simulink library "AEMS_Standard_Library"  (R2016b)
settings: Solver=ode45  StartTime=0.0  StopTime=10.0  RelTol=1e-3
undefined symbols (not defined in the file or in its folder): BkPY, carto, Cbx_extegr, Cbx_lpegrsys, Cbx_portegr, Cnx_bnk_nr_conf, Cnx_cyl_nr_conf, ConfigManagement, configuration_management, Cxx_dcm_io_tmr_end_xxxx, Cxx_dcm_rt_tmr_end, Cxx_DID_xxxx_IO_max, Cxx_DID_xxxx_IO_min, Cxx_egrhsofs, Cxx_vmaniegi, DEM_DEBOUNCE_FREEZE, DEM_DTR_CTL_INVISIBLE, DEM_DTR_CTL_NORMAL, Dem_DtrId2_XXX, Dem_DtrId3_XXX, Dem_DtrId4_XXX, Dem_DtrId5_XXX, Dem_DtrId6_XXX, Dem_DtrId7_XXX, Dem_DtrId8_XXX, Dem_DtrId9_XXX, Dem_DtrId_XXX, Dem_EnableConditionId2_XXX, Dem_EnableConditionId3_XXX, Dem_EnableConditionId4_XXX, Dem_EnableConditionId5_XXX, Dem_EnableConditionId6_XXX, Dem_EnableConditionId7_XXX, Dem_EnableConditionId8_XXX, Dem_EnableConditionId_XXX, Dem_EventId, Dem_EventId2_XXX, Dem_EventId3_XXX, Dem_EventId4_XXX, Dem_EventId5_XXX, Dem_EventId6_XXX, Dem_EventId7_XXX, Dem_EventId8_XXX, Dem_EventId9_XXX, Dem_EventId_Device_Faulttype, Dem_EventId_XXX, DEM_IUMPR_GENERAL_DENOMINATOR, DEM_OPCYC_IGNITION, Dem_RatioId2_XXX, Dem_RatioId3_XXX, Dem_RatioId4_XXX, Dem_RatioId5_XXX, Dem_RatioId6_XXX, Dem_RatioId7_XXX, Dem_RatioId8_XXX, Dem_RatioId_XXX, Dem_StorageConditionId2_XXX, Dem_StorageConditionId3_XXX, Dem_StorageConditionId4_XXX, Dem_StorageConditionId5_XXX ... (+65)
libraries: AEMS_Standard_Library x477, simulink x2
(part 24 of 39)

== system AEMS_Standard_Library/SUB/AEMS_DEM_SET_STORAGE_COND_8D ==
  conditionfulfilled : Inport
  AEMS_DEM_SETENABLECONDITION{1..8} (8 alike) : AEMS_Standard_Library/SUB/AEMS_DEM_SETENABLECONDITION  Tag=[LIB]
      settings: AttributesFormatString=%<MaskType>
  Demux2 : Demux  Outputs=8
  StorageConditionId_block1 : Constant  Value=Dem_StorageConditionId_XXX  OutDataTypeStr=uint8
  StorageConditionId_block2 : Constant  Value=Dem_StorageConditionId2_XXX  OutDataTypeStr=uint8
  StorageConditionId_block3 : Constant  Value=Dem_StorageConditionId3_XXX  OutDataTypeStr=uint8
  StorageConditionId_block4 : Constant  Value=Dem_StorageConditionId4_XXX  OutDataTypeStr=uint8
  StorageConditionId_block5 : Constant  Value=Dem_StorageConditionId5_XXX  OutDataTypeStr=uint8
  StorageConditionId_block6 : Constant  Value=Dem_StorageConditionId6_XXX  OutDataTypeStr=uint8
  StorageConditionId_block7 : Constant  Value=Dem_StorageConditionId7_XXX  OutDataTypeStr=uint8
  StorageConditionId_block8 : Constant  Value=Dem_StorageConditionId8_XXX  OutDataTypeStr=uint8
  wires:
  conditionfulfilled/1 -> Demux2/1  "conditionfulfilled"
  StorageConditionId_block1/1 -> AEMS_DEM_SETENABLECONDITION1/1  "storageconditionid1"
  StorageConditionId_block2/1 -> AEMS_DEM_SETENABLECONDITION2/1  "storageconditionid2"
  StorageConditionId_block4/1 -> AEMS_DEM_SETENABLECONDITION4/1  "storageconditionid4"
  StorageConditionId_block5/1 -> AEMS_DEM_SETENABLECONDITION5/1  "storageconditionid5"
  StorageConditionId_block3/1 -> AEMS_DEM_SETENABLECONDITION3/1  "storageconditionid3"
  StorageConditionId_block6/1 -> AEMS_DEM_SETENABLECONDITION6/1  "storageconditionid6"
  StorageConditionId_block7/1 -> AEMS_DEM_SETENABLECONDITION7/1  "storageconditionid7"
  StorageConditionId_block8/1 -> AEMS_DEM_SETENABLECONDITION8/1  "storageconditionid8"
  Demux2/1 -> AEMS_DEM_SETENABLECONDITION1/2  "conditionfulfilled1"
  Demux2/2 -> AEMS_DEM_SETENABLECONDITION2/2  "conditionfulfilled2"
  Demux2/3 -> AEMS_DEM_SETENABLECONDITION3/2  "conditionfulfilled3"
  Demux2/4 -> AEMS_DEM_SETENABLECONDITION4/2  "conditionfulfilled4"
  Demux2/5 -> AEMS_DEM_SETENABLECONDITION5/2  "conditionfulfilled5"
  Demux2/6 -> AEMS_DEM_SETENABLECONDITION6/2  "conditionfulfilled6"
  Demux2/7 -> AEMS_DEM_SETENABLECONDITION7/2  "conditionfulfilled7"
  Demux2/8 -> AEMS_DEM_SETENABLECONDITION8/2  "conditionfulfilled8"

== system AEMS_Standard_Library/SUB/AEMS_DEM_TIMEBASEDDEBOUNCE ==
  conditionfulfilled : Inport  OutDataTypeStr=boolean
  prefailed : Inport  Port=2  OutDataTypeStr=boolean
  prepassed : Inport  Port=3  OutDataTypeStr=boolean
  behavior : Inport  Port=4  OutDataTypeStr=uint8
  failedthreshold : Inport  Port=5  OutDataTypeStr=single
  passedthreshold : Inport  Port=6  OutDataTypeStr=single
  reseteventdebounce : Inport  Port=7  OutDataTypeStr=boolean
  Dem_SetEventStatus_Call : Subsystem  TreatAsAtomicUnit=on
  Subsystem_Timer_Debounce_Call : Subsystem
  debouncevalue_for_failed : Outport
  debouncevalue_for_passed : Outport  Port=2
  failed : Outport  Port=3
  passed : Outport  Port=4
  wires:
  Subsystem_Timer_Debounce_Call/6(eventstatus) -> Dem_SetEventStatus_Call/1(event_status)
  Subsystem_Timer_Debounce_Call/5(call_seteventstatus) -> Dem_SetEventStatus_Call/Enable
  Subsystem_Timer_Debounce_Call/1(debouncevalue_for_failed) -> debouncevalue_for_failed/1
  Subsystem_Timer_Debounce_Call/2(debouncevalue_for_passed) -> debouncevalue_for_passed/1
  Subsystem_Timer_Debounce_Call/3(failed) -> failed/1
  Subsystem_Timer_Debounce_Call/4(passed) -> passed/1
  conditionfulfilled/1 -> Subsystem_Timer_Debounce_Call/1(conditionfulfilled)
  prefailed/1 -> Subsystem_Timer_Debounce_Call/2(prefailed)
  prepassed/1 -> Subsystem_Timer_Debounce_Call/3(prepassed)
  behavior/1 -> Subsystem_Timer_Debounce_Call/4(behavior)
  failedthreshold/1 -> Subsystem_Timer_Debounce_Call/5(failedthreshold)
  passedthreshold/1 -> Subsystem_Timer_Debounce_Call/6(passedthreshold)
  reseteventdebounce/1 -> Subsystem_Timer_Debounce_Call/7(reseteventdebounce)

== system AEMS_Standard_Library/SUB/AEMS_DEM_TIME_BASED_DEBOUNCE_1D ==
  note: DemDebounceBehavior
  flag_set : Inport
  conditionfulfilled : Inport  Port=2
  prefailed : Inport  Port=3
  prepassed : Inport  Port=4
  reseteventdebounce : Inport  Port=5
  AEMS_DEM_TIME_BASED_DEBOUNCE_CALL : Subsystem
  DemCounterFailedThreshold : Constant  Value=DemDebounceTimeFailedThreshold
  DemCounterPassedThreshold : Constant  Value=DemDebounceTimePassedThreshold
  DemDebounceBehavior : Constant  Value=0  OutDataTypeStr=uint8
  debouncevalue_for_failed : Outport
  debouncevalue_for_passed : Outport  Port=2
  failed : Outport  Port=3
  passed : Outport  Port=4
  wires:
  conditionfulfilled/1 -> AEMS_DEM_TIME_BASED_DEBOUNCE_CALL/1(conditionfulfilled)  "conditionfulfilled"
  prefailed/1 -> AEMS_DEM_TIME_BASED_DEBOUNCE_CALL/2(prefailed)  "prefailed"
  prepassed/1 -> AEMS_DEM_TIME_BASED_DEBOUNCE_CALL/3(prepassed)  "prepassed"
  reseteventdebounce/1 -> AEMS_DEM_TIME_BASED_DEBOUNCE_CALL/4(reseteventdebounce)  "reseteventdebounce"
  DemDebounceBehavior/1 -> AEMS_DEM_TIME_BASED_DEBOUNCE_CALL/5(DemDebounceBehavior)  "behavior"
  DemCounterFailedThreshold/1 -> AEMS_DEM_TIME_BASED_DEBOUNCE_CALL/6(DemCounterFailedThreshold)  "failedthreshold"
  DemCounterPassedThreshold/1 -> AEMS_DEM_TIME_BASED_DEBOUNCE_CALL/7(DemCounterPassedThreshold)  "passedthreshold"
  AEMS_DEM_TIME_BASED_DEBOUNCE_CALL/1(debouncevalue_for_failed) -> debouncevalue_for_failed/1
  AEMS_DEM_TIME_BASED_DEBOUNCE_CALL/2(debouncevalue_for_passed) -> debouncevalue_for_passed/1
  AEMS_DEM_TIME_BASED_DEBOUNCE_CALL/3(failed) -> failed/1
  AEMS_DEM_TIME_BASED_DEBOUNCE_CALL/4(passed) -> passed/1
  flag_set/1 -> AEMS_DEM_TIME_BASED_DEBOUNCE_CALL/Enable

== system AEMS_Standard_Library/SUB/AEMS_DEM_TIME_BASED_DEBOUNCE_2D ==
  note: DemDebounceBehavior
  flag_set : Inport
  conditionfulfilled : Inport  Port=2
  prefailed : Inport  Port=3
  prepassed : Inport  Port=4
  reseteventdebounce : Inport  Port=5
  AEMS_DEM_TIME_BASED_DEBOUNCE_CALL1 : Subsystem
  AEMS_DEM_TIME_BASED_DEBOUNCE_CALL2 : Subsystem
  DemCounterFailedThreshold : Constant  Value=DemDebounceTimeFailedThreshold
  DemCounterPassedThreshold : Constant  Value=DemDebounceTimePassedThreshold
  DemDebounceBehavior : Constant  Value=[0,0]  OutDataTypeStr=uint8
  Demux{,1..7} (8 alike) : Demux  Outputs=2
  Mux{1..4} (4 alike) : Mux  Inputs=2
  debouncevalue_for_failed : Outport
  debouncevalue_for_passed : Outport  Port=2
  failed : Outport  Port=3
  passed : Outport  Port=4
  wires:
  AEMS_DEM_TIME_BASED_DEBOUNCE_CALL2/4(passed) -> Mux4/2
  Mux4/1 -> passed/1
  AEMS_DEM_TIME_BASED_DEBOUNCE_CALL1/4(passed) -> Mux4/1
  AEMS_DEM_TIME_BASED_DEBOUNCE_CALL2/3(failed) -> Mux3/2
  AEMS_DEM_TIME_BASED_DEBOUNCE_CALL1/3(failed) -> Mux3/1
  Mux3/1 -> failed/1
  AEMS_DEM_TIME_BASED_DEBOUNCE_CALL2/2(debouncevalue_for_passed) -> Mux2/2
  AEMS_DEM_TIME_BASED_DEBOUNCE_CALL1/2(debouncevalue_for_passed) -> Mux2/1
  Mux2/1 -> debouncevalue_for_passed/1
  AEMS_DEM_TIME_BASED_DEBOUNCE_CALL2/1(debouncevalue_for_failed) -> Mux1/2
  AEMS_DEM_TIME_BASED_DEBOUNCE_CALL1/1(debouncevalue_for_failed) -> Mux1/1
  Mux1/1 -> debouncevalue_for_failed/1
  Demux7/2 -> AEMS_DEM_TIME_BASED_DEBOUNCE_CALL2/7(DemCounterPassedThreshold)
  DemCounterPassedThreshold/1 -> Demux7/1  "passedthreshold"
  Demux7/1 -> AEMS_DEM_TIME_BASED_DEBOUNCE_CALL1/7(DemCounterPassedThreshold)
  Demux6/2 -> AEMS_DEM_TIME_BASED_DEBOUNCE_CALL2/6(DemCounterFailedThreshold)
  DemCounterFailedThreshold/1 -> Demux6/1  "failedthreshold"
  Demux6/1 -> AEMS_DEM_TIME_BASED_DEBOUNCE_CALL1/6(DemCounterFailedThreshold)
  Demux5/2 -> AEMS_DEM_TIME_BASED_DEBOUNCE_CALL2/5(DemDebounceBehavior)
  Demux5/1 -> AEMS_DEM_TIME_BASED_DEBOUNCE_CALL1/5(DemDebounceBehavior)
  DemDebounceBehavior/1 -> Demux5/1  "behavior"
  Demux4/2 -> AEMS_DEM_TIME_BASED_DEBOUNCE_CALL2/4(reseteventdebounce)
  reseteventdebounce/1 -> Demux4/1  "reseteventdebounce"
  Demux4/1 -> AEMS_DEM_TIME_BASED_DEBOUNCE_CALL1/4(reseteventdebounce)
  Demux3/2 -> AEMS_DEM_TIME_BASED_DEBOUNCE_CALL2/3(prepassed)
  Demux3/1 -> AEMS_DEM_TIME_BASED_DEBOUNCE_CALL1/3(prepassed)
  prepassed/1 -> Demux3/1  "prepassed"
  Demux2/2 -> AEMS_DEM_TIME_BASED_DEBOUNCE_CALL2/2(prefailed)
  Demux2/1 -> AEMS_DEM_TIME_BASED_DEBOUNCE_CALL1/2(prefailed)
  prefailed/1 -> Demux2/1  "prefailed"
  Demux1/2 -> AEMS_DEM_TIME_BASED_DEBOUNCE_CALL2/1(conditionfulfilled)
  Demux/2 -> AEMS_DEM_TIME_BASED_DEBOUNCE_CALL2/Enable
  Demux1/1 -> AEMS_DEM_TIME_BASED_DEBOUNCE_CALL1/1(conditionfulfilled)
  conditionfulfilled/1 -> Demux1/1  "conditionfulfilled"
  Demux/1 -> AEMS_DEM_TIME_BASED_DEBOUNCE_CALL1/Enable
  flag_set/1 -> Demux/1

== system AEMS_Standard_Library/SUB/AEMS_DEM_TIME_BASED_DEBOUNCE_3D ==
  note: DemDebounceBehavior
  flag_set : Inport
  conditionfulfilled : Inport  Port=2
  prefailed : Inport  Port=3
  prepassed : Inport  Port=4
  reseteventdebounce : Inport  Port=5
  AEMS_DEM_TIME_BASED_DEBOUNCE_CALL1 : Subsystem
  AEMS_DEM_TIME_BASED_DEBOUNCE_CALL2 : Subsystem
  AEMS_DEM_TIME_BASED_DEBOUNCE_CALL3 : Subsystem
  DemCounterFailedThreshold : Constant  Value=DemDebounceTimeFailedThreshold
  DemCounterPassedThreshold : Constant  Value=DemDebounceTimePassedThreshold
  DemDebounceBehavior : Constant  Value=[0,0,0]  OutDataTypeStr=uint8
  Demux{,1..7} (8 alike) : Demux  Outputs=3
  Mux{1..4} (4 alike) : Mux  Inputs=3
  debouncevalue_for_failed : Outport
  debouncevalue_for_passed : Outport  Port=2
  failed : Outport  Port=3
  passed : Outport  Port=4
  wires:
  AEMS_DEM_TIME_BASED_DEBOUNCE_CALL3/4(passed) -> Mux4/3
  AEMS_DEM_TIME_BASED_DEBOUNCE_CALL3/3(failed) -> Mux3/3
  AEMS_DEM_TIME_BASED_DEBOUNCE_CALL3/2(debouncevalue_for_passed) -> Mux2/3
  AEMS_DEM_TIME_BASED_DEBOUNCE_CALL3/1(debouncevalue_for_failed) -> Mux1/3
  Demux7/3 -> AEMS_DEM_TIME_BASED_DEBOUNCE_CALL3/7(DemCounterPassedThreshold)
  Demux6/3 -> AEMS_DEM_TIME_BASED_DEBOUNCE_CALL3/6(DemCounterFailedThreshold)
  Demux5/3 -> AEMS_DEM_TIME_BASED_DEBOUNCE_CALL3/5(DemDebounceBehavior)
  Demux4/3 -> AEMS_DEM_TIME_BASED_DEBOUNCE_CALL3/4(reseteventdebounce)
  Demux3/3 -> AEMS_DEM_TIME_BASED_DEBOUNCE_CALL3/3(prepassed)
  Demux2/3 -> AEMS_DEM_TIME_BASED_DEBOUNCE_CALL3/2(prefailed)
  Demux1/3 -> AEMS_DEM_TIME_BASED_DEBOUNCE_CALL3/1(conditionfulfilled)
  Demux/3 -> AEMS_DEM_TIME_BASED_DEBOUNCE_CALL3/Enable
  AEMS_DEM_TIME_BASED_DEBOUNCE_CALL2/4(passed) -> Mux4/2
  Mux4/1 -> passed/1
  AEMS_DEM_TIME_BASED_DEBOUNCE_CALL1/4(passed) -> Mux4/1
  AEMS_DEM_TIME_BASED_DEBOUNCE_CALL2/3(failed) -> Mux3/2
  AEMS_DEM_TIME_BASED_DEBOUNCE_CALL1/3(failed) -> Mux3/1
  Mux3/1 -> failed/1
  AEMS_DEM_TIME_BASED_DEBOUNCE_CALL2/2(debouncevalue_for_passed) -> Mux2/2
  AEMS_DEM_TIME_BASED_DEBOUNCE_CALL1/2(debouncevalue_for_passed) -> Mux2/1
  Mux2/1 -> debouncevalue_for_passed/1
  AEMS_DEM_TIME_BASED_DEBOUNCE_CALL2/1(debouncevalue_for_failed) -> Mux1/2
  AEMS_DEM_TIME_BASED_DEBOUNCE_CALL1/1(debouncevalue_for_failed) -> Mux1/1
  Mux1/1 -> debouncevalue_for_failed/1
  Demux7/2 -> AEMS_DEM_TIME_BASED_DEBOUNCE_CALL2/7(DemCounterPassedThreshold)
  DemCounterPassedThreshold/1 -> Demux7/1  "passedthreshold"
  Demux7/1 -> AEMS_DEM_TIME_BASED_DEBOUNCE_CALL1/7(DemCounterPassedThreshold)
  Demux6/2 -> AEMS_DEM_TIME_BASED_DEBOUNCE_CALL2/6(DemCounterFailedThreshold)
  DemCounterFailedThreshold/1 -> Demux6/1  "failedthreshold"
  Demux6/1 -> AEMS_DEM_TIME_BASED_DEBOUNCE_CALL1/6(DemCounterFailedThreshold)
  Demux5/2 -> AEMS_DEM_TIME_BASED_DEBOUNCE_CALL2/5(DemDebounceBehavior)
  Demux5/1 -> AEMS_DEM_TIME_BASED_DEBOUNCE_CALL1/5(DemDebounceBehavior)
  DemDebounceBehavior/1 -> Demux5/1  "behavior"
  Demux4/2 -> AEMS_DEM_TIME_BASED_DEBOUNCE_CALL2/4(reseteventdebounce)
  reseteventdebounce/1 -> Demux4/1  "reseteventdebounce"
  Demux4/1 -> AEMS_DEM_TIME_BASED_DEBOUNCE_CALL1/4(reseteventdebounce)
  Demux3/2 -> AEMS_DEM_TIME_BASED_DEBOUNCE_CALL2/3(prepassed)
  Demux3/1 -> AEMS_DEM_TIME_BASED_DEBOUNCE_CALL1/3(prepassed)
  prepassed/1 -> Demux3/1  "prepassed"
  Demux2/2 -> AEMS_DEM_TIME_BASED_DEBOUNCE_CALL2/2(prefailed)
  Demux2/1 -> AEMS_DEM_TIME_BASED_DEBOUNCE_CALL1/2(prefailed)
  prefailed/1 -> Demux2/1  "prefailed"
  Demux1/2 -> AEMS_DEM_TIME_BASED_DEBOUNCE_CALL2/1(conditionfulfilled)
  Demux/2 -> AEMS_DEM_TIME_BASED_DEBOUNCE_CALL2/Enable
  Demux1/1 -> AEMS_DEM_TIME_BASED_DEBOUNCE_CALL1/1(conditionfulfilled)
  conditionfulfilled/1 -> Demux1/1  "conditionfulfilled"
  Demux/1 -> AEMS_DEM_TIME_BASED_DEBOUNCE_CALL1/Enable
  flag_set/1 -> Demux/1

== system AEMS_Standard_Library/SUB/AEMS_DEM_TIME_BASED_DEBOUNCE_4D ==
  note: DemDebounceBehavior
  flag_set : Inport
  conditionfulfilled : Inport  Port=2
  prefailed : Inport  Port=3
  prepassed : Inport  Port=4
  reseteventdebounce : Inport  Port=5
  AEMS_DEM_TIME_BASED_DEBOUNCE_CALL1 : Subsystem
  AEMS_DEM_TIME_BASED_DEBOUNCE_CALL2 : Subsystem
  AEMS_DEM_TIME_BASED_DEBOUNCE_CALL3 : Subsystem
  AEMS_DEM_TIME_BASED_DEBOUNCE_CALL4 : Subsystem
  DemCounterFailedThreshold : Constant  Value=DemDebounceTimeFailedThreshold
  DemCounterPassedThreshold : Constant  Value=DemDebounceTimePassedThreshold
  DemDebounceBehavior : Constant  Value=[0,0,0,0]  OutDataTypeStr=uint8
  Demux{,1..7} (8 alike) : Demux
  Mux{1..4} (4 alike) : Mux
  debouncevalue_for_failed : Outport
  debouncevalue_for_passed : Outport  Port=2
  failed : Outport  Port=3
  passed : Outport  Port=4
  wires:
  AEMS_DEM_TIME_BASED_DEBOUNCE_CALL4/4(passed) -> Mux4/4
  AEMS_DEM_TIME_BASED_DEBOUNCE_CALL4/3(failed) -> Mux3/4
  AEMS_DEM_TIME_BASED_DEBOUNCE_CALL4/2(debouncevalue_for_passed) -> Mux2/4
  AEMS_DEM_TIME_BASED_DEBOUNCE_CALL4/1(debouncevalue_for_failed) -> Mux1/4
  Demux7/4 -> AEMS_DEM_TIME_BASED_DEBOUNCE_CALL4/7(DemCounterPassedThreshold)
  Demux6/4 -> AEMS_DEM_TIME_BASED_DEBOUNCE_CALL4/6(DemCounterFailedThreshold)
  Demux5/4 -> AEMS_DEM_TIME_BASED_DEBOUNCE_CALL4/5(DemDebounceBehavior)
  Demux4/4 -> AEMS_DEM_TIME_BASED_DEBOUNCE_CALL4/4(reseteventdebounce)
  Demux3/4 -> AEMS_DEM_TIME_BASED_DEBOUNCE_CALL4/3(prepassed)
  Demux2/4 -> AEMS_DEM_TIME_BASED_DEBOUNCE_CALL4/2(prefailed)
  Demux1/4 -> AEMS_DEM_TIME_BASED_DEBOUNCE_CALL4/1(conditionfulfilled)
  Demux/4 -> AEMS_DEM_TIME_BASED_DEBOUNCE_CALL4/Enable
  AEMS_DEM_TIME_BASED_DEBOUNCE_CALL3/4(passed) -> Mux4/3
  AEMS_DEM_TIME_BASED_DEBOUNCE_CALL3/3(failed) -> Mux3/3
  AEMS_DEM_TIME_BASED_DEBOUNCE_CALL3/2(debouncevalue_for_passed) -> Mux2/3
  AEMS_DEM_TIME_BASED_DEBOUNCE_CALL3/1(debouncevalue_for_failed) -> Mux1/3
  Demux7/3 -> AEMS_DEM_TIME_BASED_DEBOUNCE_CALL3/7(DemCounterPassedThreshold)
  Demux6/3 -> AEMS_DEM_TIME_BASED_DEBOUNCE_CALL3/6(DemCounterFailedThreshold)
  Demux5/3 -> AEMS_DEM_TIME_BASED_DEBOUNCE_CALL3/5(DemDebounceBehavior)
  Demux4/3 -> AEMS_DEM_TIME_BASED_DEBOUNCE_CALL3/4(reseteventdebounce)
  Demux3/3 -> AEMS_DEM_TIME_BASED_DEBOUNCE_CALL3/3(prepassed)
  Demux2/3 -> AEMS_DEM_TIME_BASED_DEBOUNCE_CALL3/2(prefailed)
  Demux1/3 -> AEMS_DEM_TIME_BASED_DEBOUNCE_CALL3/1(conditionfulfilled)
  Demux/3 -> AEMS_DEM_TIME_BASED_DEBOUNCE_CALL3/Enable
  AEMS_DEM_TIME_BASED_DEBOUNCE_CALL2/4(passed) -> Mux4/2
  Mux4/1 -> passed/1
  AEMS_DEM_TIME_BASED_DEBOUNCE_CALL1/4(passed) -> Mux4/1
  AEMS_DEM_TIME_BASED_DEBOUNCE_CALL2/3(failed) -> Mux3/2
  AEMS_DEM_TIME_BASED_DEBOUNCE_CALL1/3(failed) -> Mux3/1
  Mux3/1 -> failed/1
  AEMS_DEM_TIME_BASED_DEBOUNCE_CALL2/2(debouncevalue_for_passed) -> Mux2/2
  AEMS_DEM_TIME_BASED_DEBOUNCE_CALL1/2(debouncevalue_for_passed) -> Mux2/1
  Mux2/1 -> debouncevalue_for_passed/1
  AEMS_DEM_TIME_BASED_DEBOUNCE_CALL2/1(debouncevalue_for_failed) -> Mux1/2
  AEMS_DEM_TIME_BASED_DEBOUNCE_CALL1/1(debouncevalue_for_failed) -> Mux1/1
  Mux1/1 -> debouncevalue_for_failed/1
  Demux7/2 -> AEMS_DEM_TIME_BASED_DEBOUNCE_CALL2/7(DemCounterPassedThreshold)
  DemCounterPassedThreshold/1 -> Demux7/1  "passedthreshold"
  Demux7/1 -> AEMS_DEM_TIME_BASED_DEBOUNCE_CALL1/7(DemCounterPassedThreshold)
  Demux6/2 -> AEMS_DEM_TIME_BASED_DEBOUNCE_CALL2/6(DemCounterFailedThreshold)
  DemCounterFailedThreshold/1 -> Demux6/1  "failedthreshold"
  Demux6/1 -> AEMS_DEM_TIME_BASED_DEBOUNCE_CALL1/6(DemCounterFailedThreshold)
  Demux5/2 -> AEMS_DEM_TIME_BASED_DEBOUNCE_CALL2/5(DemDebounceBehavior)
  Demux5/1 -> AEMS_DEM_TIME_BASED_DEBOUNCE_CALL1/5(DemDebounceBehavior)
  DemDebounceBehavior/1 -> Demux5/1  "behavior"
  Demux4/2 -> AEMS_DEM_TIME_BASED_DEBOUNCE_CALL2/4(reseteventdebounce)
  reseteventdebounce/1 -> Demux4/1  "reseteventdebounce"
  Demux4/1 -> AEMS_DEM_TIME_BASED_DEBOUNCE_CALL1/4(reseteventdebounce)
  Demux3/2 -> AEMS_DEM_TIME_BASED_DEBOUNCE_CALL2/3(prepassed)
  Demux3/1 -> AEMS_DEM_TIME_BASED_DEBOUNCE_CALL1/3(prepassed)
  prepassed/1 -> Demux3/1  "prepassed"
  Demux2/2 -> AEMS_DEM_TIME_BASED_DEBOUNCE_CALL2/2(prefailed)
  Demux2/1 -> AEMS_DEM_TIME_BASED_DEBOUNCE_CALL1/2(prefailed)
  prefailed/1 -> Demux2/1  "prefailed"
  Demux1/2 -> AEMS_DEM_TIME_BASED_DEBOUNCE_CALL2/1(conditionfulfilled)
  Demux/2 -> AEMS_DEM_TIME_BASED_DEBOUNCE_CALL2/Enable
  Demux1/1 -> AEMS_DEM_TIME_BASED_DEBOUNCE_CALL1/1(conditionfulfilled)
  conditionfulfilled/1 -> Demux1/1  "conditionfulfilled"
  Demux/1 -> AEMS_DEM_TIME_BASED_DEBOUNCE_CALL1/Enable
  flag_set/1 -> Demux/1

== system AEMS_Standard_Library/SUB/AEMS_DEM_TIME_BASED_DEBOUNCE_6D ==
  note: DemDebounceBehavior
  flag_set : Inport
  conditionfulfilled : Inport  Port=2
  prefailed : Inport  Port=3
  prepassed : Inport  Port=4
  reseteventdebounce : Inport  Port=5
  AEMS_DEM_TIME_BASED_DEBOUNCE_CALL1 : Subsystem
  AEMS_DEM_TIME_BASED_DEBOUNCE_CALL2 : Subsystem
  AEMS_DEM_TIME_BASED_DEBOUNCE_CALL3 : Subsystem
  AEMS_DEM_TIME_BASED_DEBOUNCE_CALL4 : Subsystem
  AEMS_DEM_TIME_BASED_DEBOUNCE_CALL5 : Subsystem
  AEMS_DEM_TIME_BASED_DEBOUNCE_CALL6 : Subsystem
  DemCounterFailedThreshold : Constant  Value=DemDebounceTimeFailedThreshold
  DemCounterPassedThreshold : Constant  Value=DemDebounceTimePassedThreshold
  DemDebounceBehavior : Constant  Value=[0,0,0,0,0,0]  OutDataTypeStr=uint8
  Demux{,1..7} (8 alike) : Demux  Outputs=6
  Mux{1..4} (4 alike) : Mux  Inputs=6
  debouncevalue_for_failed : Outport
  debouncevalue_for_passed : Outport  Port=2
  failed : Outport  Port=3
  passed : Outport  Port=4
  wires:
  AEMS_DEM_TIME_BASED_DEBOUNCE_CALL6/4(passed) -> Mux4/6
  AEMS_DEM_TIME_BASED_DEBOUNCE_CALL5/4(passed) -> Mux4/5
  AEMS_DEM_TIME_BASED_DEBOUNCE_CALL6/3(failed) -> Mux3/6
  AEMS_DEM_TIME_BASED_DEBOUNCE_CALL5/3(failed) -> Mux3/5
  AEMS_DEM_TIME_BASED_DEBOUNCE_CALL6/2(debouncevalue_for_passed) -> Mux2/6
  AEMS_DEM_TIME_BASED_DEBOUNCE_CALL5/2(debouncevalue_for_passed) -> Mux2/5
  AEMS_DEM_TIME_BASED_DEBOUNCE_CALL6/1(debouncevalue_for_failed) -> Mux1/6
  AEMS_DEM_TIME_BASED_DEBOUNCE_CALL5/1(debouncevalue_for_failed) -> Mux1/5
  Demux7/6 -> AEMS_DEM_TIME_BASED_DEBOUNCE_CALL6/7(DemCounterPassedThreshold)
  Demux7/5 -> AEMS_DEM_TIME_BASED_DEBOUNCE_CALL5/7(DemCounterPassedThreshold)
  Demux6/6 -> AEMS_DEM_TIME_BASED_DEBOUNCE_CALL6/6(DemCounterFailedThreshold)
  Demux6/5 -> AEMS_DEM_TIME_BASED_DEBOUNCE_CALL5/6(DemCounterFailedThreshold)
  Demux5/6 -> AEMS_DEM_TIME_BASED_DEBOUNCE_CALL6/5(DemDebounceBehavior)
  Demux5/5 -> AEMS_DEM_TIME_BASED_DEBOUNCE_CALL5/5(DemDebounceBehavior)
  Demux4/6 -> AEMS_DEM_TIME_BASED_DEBOUNCE_CALL6/4(reseteventdebounce)
  Demux4/5 -> AEMS_DEM_TIME_BASED_DEBOUNCE_CALL5/4(reseteventdebounce)
  Demux3/6 -> AEMS_DEM_TIME_BASED_DEBOUNCE_CALL6/3(prepassed)
  Demux3/5 -> AEMS_DEM_TIME_BASED_DEBOUNCE_CALL5/3(prepassed)
  Demux2/6 -> AEMS_DEM_TIME_BASED_DEBOUNCE_CALL6/2(prefailed)
  Demux2/5 -> AEMS_DEM_TIME_BASED_DEBOUNCE_CALL5/2(prefailed)
  Demux1/6 -> AEMS_DEM_TIME_BASED_DEBOUNCE_CALL6/1(conditionfulfilled)
  Demux1/5 -> AEMS_DEM_TIME_BASED_DEBOUNCE_CALL5/1(conditionfulfilled)
  Demux/6 -> AEMS_DEM_TIME_BASED_DEBOUNCE_CALL6/Enable
  Demux/5 -> AEMS_DEM_TIME_BASED_DEBOUNCE_CALL5/Enable
  AEMS_DEM_TIME_BASED_DEBOUNCE_CALL4/4(passed) -> Mux4/4
  AEMS_DEM_TIME_BASED_DEBOUNCE_CALL4/3(failed) -> Mux3/4
  AEMS_DEM_TIME_BASED_DEBOUNCE_CALL4/2(debouncevalue_for_passed) -> Mux2/4
  AEMS_DEM_TIME_BASED_DEBOUNCE_CALL4/1(debouncevalue_for_failed) -> Mux1/4
  Demux7/4 -> AEMS_DEM_TIME_BASED_DEBOUNCE_CALL4/7(DemCounterPassedThreshold)
  Demux6/4 -> AEMS_DEM_TIME_BASED_DEBOUNCE_CALL4/6(DemCounterFailedThreshold)
  Demux5/4 -> AEMS_DEM_TIME_BASED_DEBOUNCE_CALL4/5(DemDebounceBehavior)
  Demux4/4 -> AEMS_DEM_TIME_BASED_DEBOUNCE_CALL4/4(reseteventdebounce)
  Demux3/4 -> AEMS_DEM_TIME_BASED_DEBOUNCE_CALL4/3(prepassed)
  Demux2/4 -> AEMS_DEM_TIME_BASED_DEBOUNCE_CALL4/2(prefailed)
  Demux1/4 -> AEMS_DEM_TIME_BASED_DEBOUNCE_CALL4/1(conditionfulfilled)
  Demux/4 -> AEMS_DEM_TIME_BASED_DEBOUNCE_CALL4/Enable
  AEMS_DEM_TIME_BASED_DEBOUNCE_CALL3/4(passed) -> Mux4/3
  AEMS_DEM_TIME_BASED_DEBOUNCE_CALL3/3(failed) -> Mux3/3
  AEMS_DEM_TIME_BASED_DEBOUNCE_CALL3/2(debouncevalue_for_passed) -> Mux2/3
  AEMS_DEM_TIME_BASED_DEBOUNCE_CALL3/1(debouncevalue_for_failed) -> Mux1/3
  Demux7/3 -> AEMS_DEM_TIME_BASED_DEBOUNCE_CALL3/7(DemCounterPassedThreshold)
  Demux6/3 -> AEMS_DEM_TIME_BASED_DEBOUNCE_CALL3/6(DemCounterFailedThreshold)
  Demux5/3 -> AEMS_DEM_TIME_BASED_DEBOUNCE_CALL3/5(DemDebounceBehavior)
  Demux4/3 -> AEMS_DEM_TIME_BASED_DEBOUNCE_CALL3/4(reseteventdebounce)
  Demux3/3 -> AEMS_DEM_TIME_BASED_DEBOUNCE_CALL3/3(prepassed)
  Demux2/3 -> AEMS_DEM_TIME_BASED_DEBOUNCE_CALL3/2(prefailed)
  Demux1/3 -> AEMS_DEM_TIME_BASED_DEBOUNCE_CALL3/1(conditionfulfilled)
  Demux/3 -> AEMS_DEM_TIME_BASED_DEBOUNCE_CALL3/Enable
  AEMS_DEM_TIME_BASED_DEBOUNCE_CALL2/4(passed) -> Mux4/2
  Mux4/1 -> passed/1
  AEMS_DEM_TIME_BASED_DEBOUNCE_CALL1/4(passed) -> Mux4/1
  AEMS_DEM_TIME_BASED_DEBOUNCE_CALL2/3(failed) -> Mux3/2
  AEMS_DEM_TIME_BASED_DEBOUNCE_CALL1/3(failed) -> Mux3/1
  Mux3/1 -> failed/1
  AEMS_DEM_TIME_BASED_DEBOUNCE_CALL2/2(debouncevalue_for_passed) -> Mux2/2
  AEMS_DEM_TIME_BASED_DEBOUNCE_CALL1/2(debouncevalue_for_passed) -> Mux2/1
  Mux2/1 -> debouncevalue_for_passed/1
  AEMS_DEM_TIME_BASED_DEBOUNCE_CALL2/1(debouncevalue_for_failed) -> Mux1/2
  AEMS_DEM_TIME_BASED_DEBOUNCE_CALL1/1(debouncevalue_for_failed) -> Mux1/1
  Mux1/1 -> debouncevalue_for_failed/1
  Demux7/2 -> AEMS_DEM_TIME_BASED_DEBOUNCE_CALL2/7(DemCounterPassedThreshold)
  DemCounterPassedThreshold/1 -> Demux7/1  "passedthreshold"
  Demux7/1 -> AEMS_DEM_TIME_BASED_DEBOUNCE_CALL1/7(DemCounterPassedThreshold)
  Demux6/2 -> AEMS_DEM_TIME_BASED_DEBOUNCE_CALL2/6(DemCounterFailedThreshold)
  DemCounterFailedThreshold/1 -> Demux6/1  "failedthreshold"
  Demux6/1 -> AEMS_DEM_TIME_BASED_DEBOUNCE_CALL1/6(DemCounterFailedThreshold)
  Demux5/2 -> AEMS_DEM_TIME_BASED_DEBOUNCE_CALL2/5(DemDebounceBehavior)
  Demux5/1 -> AEMS_DEM_TIME_BASED_DEBOUNCE_CALL1/5(DemDebounceBehavior)
  DemDebounceBehavior/1 -> Demux5/1  "behavior"
  Demux4/2 -> AEMS_DEM_TIME_BASED_DEBOUNCE_CALL2/4(reseteventdebounce)
  reseteventdebounce/1 -> Demux4/1  "reseteventdebounce"
  Demux4/1 -> AEMS_DEM_TIME_BASED_DEBOUNCE_CALL1/4(reseteventdebounce)
  Demux3/2 -> AEMS_DEM_TIME_BASED_DEBOUNCE_CALL2/3(prepassed)
  Demux3/1 -> AEMS_DEM_TIME_BASED_DEBOUNCE_CALL1/3(prepassed)
  prepassed/1 -> Demux3/1  "prepassed"
  Demux2/2 -> AEMS_DEM_TIME_BASED_DEBOUNCE_CALL2/2(prefailed)
  Demux2/1 -> AEMS_DEM_TIME_BASED_DEBOUNCE_CALL1/2(prefailed)
  prefailed/1 -> Demux2/1  "prefailed"
  Demux1/2 -> AEMS_DEM_TIME_BASED_DEBOUNCE_CALL2/1(conditionfulfilled)
  Demux/2 -> AEMS_DEM_TIME_BASED_DEBOUNCE_CALL2/Enable
  Demux1/1 -> AEMS_DEM_TIME_BASED_DEBOUNCE_CALL1/1(conditionfulfilled)
  conditionfulfilled/1 -> Demux1/1  "conditionfulfilled"
  Demux/1 -> AEMS_DEM_TIME_BASED_DEBOUNCE_CALL1/Enable
  flag_set/1 -> Demux/1

== system AEMS_Standard_Library/SUB/AEMS_DEM_TIME_BASED_DEBOUNCE_8D ==
  note: DemDebounceBehavior
  flag_set : Inport
  conditionfulfilled : Inport  Port=2
  prefailed : Inport  Port=3
  prepassed : Inport  Port=4
  reseteventdebounce : Inport  Port=5
  AEMS_DEM_TIME_BASED_DEBOUNCE_CALL1 : Subsystem
  AEMS_DEM_TIME_BASED_DEBOUNCE_CALL2 : Subsystem
  AEMS_DEM_TIME_BASED_DEBOUNCE_CALL3 : Subsystem
  AEMS_DEM_TIME_BASED_DEBOUNCE_CALL4 : Subsystem
  AEMS_DEM_TIME_BASED_DEBOUNCE_CALL5 : Subsystem
  AEMS_DEM_TIME_BASED_DEBOUNCE_CALL6 : Subsystem
  AEMS_DEM_TIME_BASED_DEBOUNCE_CALL7 : Subsystem
  AEMS_DEM_TIME_BASED_DEBOUNCE_CALL8 : Subsystem
  DemCounterFailedThreshold : Constant  Value=DemDebounceTimeFailedThreshold
  DemCounterPassedThreshold : Constant  Value=DemDebounceTimePassedThreshold
  DemDebounceBehavior : Constant  Value=[0,0,0,0,0,0,0,0]  OutDataTypeStr=uint8
  Demux{,1..7} (8 alike) : Demux  Outputs=8
  Mux{1..4} (4 alike) : Mux  Inputs=8
  debouncevalue_for_failed : Outport
  debouncevalue_for_passed : Outport  Port=2
  failed : Outport  Port=3
  passed : Outport  Port=4
  wires:
  AEMS_DEM_TIME_BASED_DEBOUNCE_CALL8/4(passed) -> Mux4/8
  AEMS_DEM_TIME_BASED_DEBOUNCE_CALL7/4(passed) -> Mux4/7
  AEMS_DEM_TIME_BASED_DEBOUNCE_CALL8/3(failed) -> Mux3/8
  AEMS_DEM_TIME_BASED_DEBOUNCE_CALL7/3(failed) -> Mux3/7
  AEMS_DEM_TIME_BASED_DEBOUNCE_CALL8/2(debouncevalue_for_passed) -> Mux2/8
  AEMS_DEM_TIME_BASED_DEBOUNCE_CALL7/2(debouncevalue_for_passed) -> Mux2/7
  AEMS_DEM_TIME_BASED_DEBOUNCE_CALL8/1(debouncevalue_for_failed) -> Mux1/8
  AEMS_DEM_TIME_BASED_DEBOUNCE_CALL7/1(debouncevalue_for_failed) -> Mux1/7
  Demux7/8 -> AEMS_DEM_TIME_BASED_DEBOUNCE_CALL8/7(DemCounterPassedThreshold)
  Demux7/7 -> AEMS_DEM_TIME_BASED_DEBOUNCE_CALL7/7(DemCounterPassedThreshold)
  Demux6/8 -> AEMS_DEM_TIME_BASED_DEBOUNCE_CALL8/6(DemCounterFailedThreshold)
  Demux6/7 -> AEMS_DEM_TIME_BASED_DEBOUNCE_CALL7/6(DemCounterFailedThreshold)
  Demux5/8 -> AEMS_DEM_TIME_BASED_DEBOUNCE_CALL8/5(DemDebounceBehavior)
  Demux5/7 -> AEMS_DEM_TIME_BASED_DEBOUNCE_CALL7/5(DemDebounceBehavior)
  Demux4/8 -> AEMS_DEM_TIME_BASED_DEBOUNCE_CALL8/4(reseteventdebounce)
  Demux4/7 -> AEMS_DEM_TIME_BASED_DEBOUNCE_CALL7/4(reseteventdebounce)
  Demux3/8 -> AEMS_DEM_TIME_BASED_DEBOUNCE_CALL8/3(prepassed)
  Demux3/7 -> AEMS_DEM_TIME_BASED_DEBOUNCE_CALL7/3(prepassed)
  Demux2/8 -> AEMS_DEM_TIME_BASED_DEBOUNCE_CALL8/2(prefailed)
  Demux2/7 -> AEMS_DEM_TIME_BASED_DEBOUNCE_CALL7/2(prefailed)
  Demux1/8 -> AEMS_DEM_TIME_BASED_DEBOUNCE_CALL8/1(conditionfulfilled)
  Demux1/7 -> AEMS_DEM_TIME_BASED_DEBOUNCE_CALL7/1(conditionfulfilled)
  Demux/8 -> AEMS_DEM_TIME_BASED_DEBOUNCE_CALL8/Enable
  Demux/7 -> AEMS_DEM_TIME_BASED_DEBOUNCE_CALL7/Enable
  AEMS_DEM_TIME_BASED_DEBOUNCE_CALL6/4(passed) -> Mux4/6
  AEMS_DEM_TIME_BASED_DEBOUNCE_CALL5/4(passed) -> Mux4/5
  AEMS_DEM_TIME_BASED_DEBOUNCE_CALL6/3(failed) -> Mux3/6
  AEMS_DEM_TIME_BASED_DEBOUNCE_CALL5/3(failed) -> Mux3/5
  AEMS_DEM_TIME_BASED_DEBOUNCE_CALL6/2(debouncevalue_for_passed) -> Mux2/6
  AEMS_DEM_TIME_BASED_DEBOUNCE_CALL5/2(debouncevalue_for_passed) -> Mux2/5
  AEMS_DEM_TIME_BASED_DEBOUNCE_CALL6/1(debouncevalue_for_failed) -> Mux1/6
  AEMS_DEM_TIME_BASED_DEBOUNCE_CALL5/1(debouncevalue_for_failed) -> Mux1/5
  Demux7/6 -> AEMS_DEM_TIME_BASED_DEBOUNCE_CALL6/7(DemCounterPassedThreshold)
  Demux7/5 -> AEMS_DEM_TIME_BASED_DEBOUNCE_CALL5/7(DemCounterPassedThreshold)
  Demux6/6 -> AEMS_DEM_TIME_BASED_DEBOUNCE_CALL6/6(DemCounterFailedThreshold)
  Demux6/5 -> AEMS_DEM_TIME_BASED_DEBOUNCE_CALL5/6(DemCounterFailedThreshold)
  Demux5/6 -> AEMS_DEM_TIME_BASED_DEBOUNCE_CALL6/5(DemDebounceBehavior)
  Demux5/5 -> AEMS_DEM_TIME_BASED_DEBOUNCE_CALL5/5(DemDebounceBehavior)
  Demux4/6 -> AEMS_DEM_TIME_BASED_DEBOUNCE_CALL6/4(reseteventdebounce)
  Demux4/5 -> AEMS_DEM_TIME_BASED_DEBOUNCE_CALL5/4(reseteventdebounce)
  Demux3/6 -> AEMS_DEM_TIME_BASED_DEBOUNCE_CALL6/3(prepassed)
  Demux3/5 -> AEMS_DEM_TIME_BASED_DEBOUNCE_CALL5/3(prepassed)
  Demux2/6 -> AEMS_DEM_TIME_BASED_DEBOUNCE_CALL6/2(prefailed)
  Demux2/5 -> AEMS_DEM_TIME_BASED_DEBOUNCE_CALL5/2(prefailed)
  Demux1/6 -> AEMS_DEM_TIME_BASED_DEBOUNCE_CALL6/1(conditionfulfilled)
  Demux1/5 -> AEMS_DEM_TIME_BASED_DEBOUNCE_CALL5/1(conditionfulfilled)
  Demux/6 -> AEMS_DEM_TIME_BASED_DEBOUNCE_CALL6/Enable
  Demux/5 -> AEMS_DEM_TIME_BASED_DEBOUNCE_CALL5/Enable
  AEMS_DEM_TIME_BASED_DEBOUNCE_CALL4/4(passed) -> Mux4/4
  AEMS_DEM_TIME_BASED_DEBOUNCE_CALL4/3(failed) -> Mux3/4
  AEMS_DEM_TIME_BASED_DEBOUNCE_CALL4/2(debouncevalue_for_passed) -> Mux2/4
  AEMS_DEM_TIME_BASED_DEBOUNCE_CALL4/1(debouncevalue_for_failed) -> Mux1/4
  Demux7/4 -> AEMS_DEM_TIME_BASED_DEBOUNCE_CALL4/7(DemCounterPassedThreshold)
  Demux6/4 -> AEMS_DEM_TIME_BASED_DEBOUNCE_CALL4/6(DemCounterFailedThreshold)
  Demux5/4 -> AEMS_DEM_TIME_BASED_DEBOUNCE_CALL4/5(DemDebounceBehavior)
  Demux4/4 -> AEMS_DEM_TIME_BASED_DEBOUNCE_CALL4/4(reseteventdebounce)
  Demux3/4 -> AEMS_DEM_TIME_BASED_DEBOUNCE_CALL4/3(prepassed)
  Demux2/4 -> AEMS_DEM_TIME_BASED_DEBOUNCE_CALL4/2(prefailed)
  Demux1/4 -> AEMS_DEM_TIME_BASED_DEBOUNCE_CALL4/1(conditionfulfilled)
  Demux/4 -> AEMS_DEM_TIME_BASED_DEBOUNCE_CALL4/Enable
  AEMS_DEM_TIME_BASED_DEBOUNCE_CALL3/4(passed) -> Mux4/3
  AEMS_DEM_TIME_BASED_DEBOUNCE_CALL3/3(failed) -> Mux3/3
  AEMS_DEM_TIME_BASED_DEBOUNCE_CALL3/2(debouncevalue_for_passed) -> Mux2/3
  AEMS_DEM_TIME_BASED_DEBOUNCE_CALL3/1(debouncevalue_for_failed) -> Mux1/3
  Demux7/3 -> AEMS_DEM_TIME_BASED_DEBOUNCE_CALL3/7(DemCounterPassedThreshold)
  Demux6/3 -> AEMS_DEM_TIME_BASED_DEBOUNCE_CALL3/6(DemCounterFailedThreshold)
  Demux5/3 -> AEMS_DEM_TIME_BASED_DEBOUNCE_CALL3/5(DemDebounceBehavior)
  Demux4/3 -> AEMS_DEM_TIME_BASED_DEBOUNCE_CALL3/4(reseteventdebounce)
  Demux3/3 -> AEMS_DEM_TIME_BASED_DEBOUNCE_CALL3/3(prepassed)
  Demux2/3 -> AEMS_DEM_TIME_BASED_DEBOUNCE_CALL3/2(prefailed)
  Demux1/3 -> AEMS_DEM_TIME_BASED_DEBOUNCE_CALL3/1(conditionfulfilled)
  Demux/3 -> AEMS_DEM_TIME_BASED_DEBOUNCE_CALL3/Enable
  AEMS_DEM_TIME_BASED_DEBOUNCE_CALL2/4(passed) -> Mux4/2
  Mux4/1 -> passed/1
  AEMS_DEM_TIME_BASED_DEBOUNCE_CALL1/4(passed) -> Mux4/1
  AEMS_DEM_TIME_BASED_DEBOUNCE_CALL2/3(failed) -> Mux3/2
  AEMS_DEM_TIME_BASED_DEBOUNCE_CALL1/3(failed) -> Mux3/1
  Mux3/1 -> failed/1
  AEMS_DEM_TIME_BASED_DEBOUNCE_CALL2/2(debouncevalue_for_passed) -> Mux2/2
  AEMS_DEM_TIME_BASED_DEBOUNCE_CALL1/2(debouncevalue_for_passed) -> Mux2/1
  Mux2/1 -> debouncevalue_for_passed/1
  AEMS_DEM_TIME_BASED_DEBOUNCE_CALL2/1(debouncevalue_for_failed) -> Mux1/2
  AEMS_DEM_TIME_BASED_DEBOUNCE_CALL1/1(debouncevalue_for_failed) -> Mux1/1
  Mux1/1 -> debouncevalue_for_failed/1
  Demux7/2 -> AEMS_DEM_TIME_BASED_DEBOUNCE_CALL2/7(DemCounterPassedThreshold)
  DemCounterPassedThreshold/1 -> Demux7/1  "passedthreshold"
  Demux7/1 -> AEMS_DEM_TIME_BASED_DEBOUNCE_CALL1/7(DemCounterPassedThreshold)
  Demux6/2 -> AEMS_DEM_TIME_BASED_DEBOUNCE_CALL2/6(DemCounterFailedThreshold)
  DemCounterFailedThreshold/1 -> Demux6/1  "failedthreshold"
  Demux6/1 -> AEMS_DEM_TIME_BASED_DEBOUNCE_CALL1/6(DemCounterFailedThreshold)
  Demux5/2 -> AEMS_DEM_TIME_BASED_DEBOUNCE_CALL2/5(DemDebounceBehavior)
  Demux5/1 -> AEMS_DEM_TIME_BASED_DEBOUNCE_CALL1/5(DemDebounceBehavior)
  DemDebounceBehavior/1 -> Demux5/1  "behavior"
  Demux4/2 -> AEMS_DEM_TIME_BASED_DEBOUNCE_CALL2/4(reseteventdebounce)
  reseteventdebounce/1 -> Demux4/1  "reseteventdebounce"
  Demux4/1 -> AEMS_DEM_TIME_BASED_DEBOUNCE_CALL1/4(reseteventdebounce)
  Demux3/2 -> AEMS_DEM_TIME_BASED_DEBOUNCE_CALL2/3(prepassed)
  Demux3/1 -> AEMS_DEM_TIME_BASED_DEBOUNCE_CALL1/3(prepassed)
  prepassed/1 -> Demux3/1  "prepassed"
  Demux2/2 -> AEMS_DEM_TIME_BASED_DEBOUNCE_CALL2/2(prefailed)
  Demux2/1 -> AEMS_DEM_TIME_BASED_DEBOUNCE_CALL1/2(prefailed)
  prefailed/1 -> Demux2/1  "prefailed"
  Demux1/2 -> AEMS_DEM_TIME_BASED_DEBOUNCE_CALL2/1(conditionfulfilled)
  Demux/2 -> AEMS_DEM_TIME_BASED_DEBOUNCE_CALL2/Enable
  Demux1/1 -> AEMS_DEM_TIME_BASED_DEBOUNCE_CALL1/1(conditionfulfilled)
  conditionfulfilled/1 -> Demux1/1  "conditionfulfilled"
  Demux/1 -> AEMS_DEM_TIME_BASED_DEBOUNCE_CALL1/Enable
  flag_set/1 -> Demux/1

== system AEMS_Standard_Library/SUB/AEMS_DEM_TIME_BASED_DEBOUNCE_THRSHOLD_DYN_1D ==
  note: DemDebounceBehavior
  flag_set : Inport
  conditionfulfilled : Inport  Port=2
  prefailed : Inport  Port=3
  prepassed : Inport  Port=4
  reseteventdebounce : Inport  Port=5
  failedthreshold : Inport  Port=6
  passedthreshold : Inport  Port=7
  AEMS_DEM_TIME_BASED_DEBOUNCE_THRSHOLD_DYN_CALL : Subsystem
  DemDebounceBehavior : Constant  Value=0  OutDataTypeStr=uint8
  debouncevalue_for_failed : Outport
  debouncevalue_for_passed : Outport  Port=2
  failed : Outport  Port=3
  passed : Outport  Port=4
  wires:
  flag_set/1 -> AEMS_DEM_TIME_BASED_DEBOUNCE_THRSHOLD_DYN_CALL/Enable
  AEMS_DEM_TIME_BASED_DEBOUNCE_THRSHOLD_DYN_CALL/4(passed) -> passed/1
  AEMS_DEM_TIME_BASED_DEBOUNCE_THRSHOLD_DYN_CALL/3(failed) -> failed/1
  AEMS_DEM_TIME_BASED_DEBOUNCE_THRSHOLD_DYN_CALL/2(debouncevalue_for_passed) -> debouncevalue_for_passed/1
  AEMS_DEM_TIME_BASED_DEBOUNCE_THRSHOLD_DYN_CALL/1(debouncevalue_for_failed) -> debouncevalue_for_failed/1
  passedthreshold/1 -> AEMS_DEM_TIME_BASED_DEBOUNCE_THRSHOLD_DYN_CALL/7(DemCounterPassedThreshold)  "passedthreshold"
  failedthreshold/1 -> AEMS_DEM_TIME_BASED_DEBOUNCE_THRSHOLD_DYN_CALL/6(DemCounterFailedThreshold)  "failedthreshold"
  DemDebounceBehavior/1 -> AEMS_DEM_TIME_BASED_DEBOUNCE_THRSHOLD_DYN_CALL/5(DemDebounceBehavior)  "behavior"
  reseteventdebounce/1 -> AEMS_DEM_TIME_BASED_DEBOUNCE_THRSHOLD_DYN_CALL/4(reseteventdebounce)  "reseteventdebounce"
  prepassed/1 -> AEMS_DEM_TIME_BASED_DEBOUNCE_THRSHOLD_DYN_CALL/3(prepassed)  "prepassed"
  prefailed/1 -> AEMS_DEM_TIME_BASED_DEBOUNCE_THRSHOLD_DYN_CALL/2(prefailed)  "prefailed"
  conditionfulfilled/1 -> AEMS_DEM_TIME_BASED_DEBOUNCE_THRSHOLD_DYN_CALL/1(conditionfulfilled)  "conditionfulfilled"

== system AEMS_Standard_Library/SUB/AEMS_DEM_TIME_BASED_DEBOUNCE_THRSHOLD_DYN_2D ==
  note: DemDebounceBehavior
  flag_set : Inport
  conditionfulfilled : Inport  Port=2
  prefailed : Inport  Port=3
  prepassed : Inport  Port=4
  reseteventdebounce : Inport  Port=5
  failedthreshold : Inport  Port=6
  passedthreshold : Inport  Port=7
  AEMS_DEM_TIME_BASED_DEBOUNCE_THRSHOLD_DYN_CALL1 : Subsystem
  AEMS_DEM_TIME_BASED_DEBOUNCE_THRSHOLD_DYN_CALL2 : Subsystem
  DemDebounceBehavior : Constant  Value=[0,0]  OutDataTypeStr=uint8
  Demux{,1..7} (8 alike) : Demux  Outputs=2
  Mux{1..4} (4 alike) : Mux  Inputs=2
  debouncevalue_for_failed : Outport
  debouncevalue_for_passed : Outport  Port=2
  failed : Outport  Port=3
  passed : Outport  Port=4
  wires:
  AEMS_DEM_TIME_BASED_DEBOUNCE_THRSHOLD_DYN_CALL2/4(passed) -> Mux4/2
  Mux4/1 -> passed/1
  AEMS_DEM_TIME_BASED_DEBOUNCE_THRSHOLD_DYN_CALL1/4(passed) -> Mux4/1
  AEMS_DEM_TIME_BASED_DEBOUNCE_THRSHOLD_DYN_CALL2/3(failed) -> Mux3/2
  AEMS_DEM_TIME_BASED_DEBOUNCE_THRSHOLD_DYN_CALL1/3(failed) -> Mux3/1
  Mux3/1 -> failed/1
  AEMS_DEM_TIME_BASED_DEBOUNCE_THRSHOLD_DYN_CALL2/2(debouncevalue_for_passed) -> Mux2/2
  AEMS_DEM_TIME_BASED_DEBOUNCE_THRSHOLD_DYN_CALL1/2(debouncevalue_for_passed) -> Mux2/1
  Mux2/1 -> debouncevalue_for_passed/1
  AEMS_DEM_TIME_BASED_DEBOUNCE_THRSHOLD_DYN_CALL2/1(debouncevalue_for_failed) -> Mux1/2
  AEMS_DEM_TIME_BASED_DEBOUNCE_THRSHOLD_DYN_CALL1/1(debouncevalue_for_failed) -> Mux1/1
  Mux1/1 -> debouncevalue_for_failed/1
  Demux7/2 -> AEMS_DEM_TIME_BASED_DEBOUNCE_THRSHOLD_DYN_CALL2/7(DemCounterPassedThreshold)
  passedthreshold/1 -> Demux7/1  "passedthreshold"
  Demux7/1 -> AEMS_DEM_TIME_BASED_DEBOUNCE_THRSHOLD_DYN_CALL1/7(DemCounterPassedThreshold)
  Demux6/2 -> AEMS_DEM_TIME_BASED_DEBOUNCE_THRSHOLD_DYN_CALL2/6(DemCounterFailedThreshold)
  failedthreshold/1 -> Demux6/1  "failedthreshold"
  Demux6/1 -> AEMS_DEM_TIME_BASED_DEBOUNCE_THRSHOLD_DYN_CALL1/6(DemCounterFailedThreshold)
  Demux5/2 -> AEMS_DEM_TIME_BASED_DEBOUNCE_THRSHOLD_DYN_CALL2/5(DemDebounceBehavior)
  Demux5/1 -> AEMS_DEM_TIME_BASED_DEBOUNCE_THRSHOLD_DYN_CALL1/5(DemDebounceBehavior)
  DemDebounceBehavior/1 -> Demux5/1  "behavior"
  Demux4/2 -> AEMS_DEM_TIME_BASED_DEBOUNCE_THRSHOLD_DYN_CALL2/4(reseteventdebounce)
  reseteventdebounce/1 -> Demux4/1  "reseteventdebounce"
  Demux4/1 -> AEMS_DEM_TIME_BASED_DEBOUNCE_THRSHOLD_DYN_CALL1/4(reseteventdebounce)
  Demux3/2 -> AEMS_DEM_TIME_BASED_DEBOUNCE_THRSHOLD_DYN_CALL2/3(prepassed)
  Demux3/1 -> AEMS_DEM_TIME_BASED_DEBOUNCE_THRSHOLD_DYN_CALL1/3(prepassed)
  prepassed/1 -> Demux3/1  "prepassed"
  Demux2/2 -> AEMS_DEM_TIME_BASED_DEBOUNCE_THRSHOLD_DYN_CALL2/2(prefailed)
  Demux2/1 -> AEMS_DEM_TIME_BASED_DEBOUNCE_THRSHOLD_DYN_CALL1/2(prefailed)
  prefailed/1 -> Demux2/1  "prefailed"
  Demux1/2 -> AEMS_DEM_TIME_BASED_DEBOUNCE_THRSHOLD_DYN_CALL2/1(conditionfulfilled)
  Demux/2 -> AEMS_DEM_TIME_BASED_DEBOUNCE_THRSHOLD_DYN_CALL2/Enable
  Demux1/1 -> AEMS_DEM_TIME_BASED_DEBOUNCE_THRSHOLD_DYN_CALL1/1(conditionfulfilled)
  conditionfulfilled/1 -> Demux1/1  "conditionfulfilled"
  Demux/1 -> AEMS_DEM_TIME_BASED_DEBOUNCE_THRSHOLD_DYN_CALL1/Enable
  flag_set/1 -> Demux/1

== system AEMS_Standard_Library/SUB/AEMS_DEM_TIME_BASED_DEBOUNCE_THRSHOLD_DYN_3D ==
  note: DemDebounceBehavior
  flag_set : Inport
  conditionfulfilled : Inport  Port=2
  prefailed : Inport  Port=3
  prepassed : Inport  Port=4
  reseteventdebounce : Inport  Port=5
  failedthreshold : Inport  Port=6
  passedthreshold : Inport  Port=7
  AEMS_DEM_TIME_BASED_DEBOUNCE_THRSHOLD_DYN_CALL1 : Subsystem
  AEMS_DEM_TIME_BASED_DEBOUNCE_THRSHOLD_DYN_CALL2 : Subsystem
  AEMS_DEM_TIME_BASED_DEBOUNCE_THRSHOLD_DYN_CALL3 : Subsystem
  DemDebounceBehavior : Constant  Value=[0,0,0]  OutDataTypeStr=uint8
  Demux{,1..7} (8 alike) : Demux  Outputs=3
  Mux{1..4} (4 alike) : Mux  Inputs=3
  debouncevalue_for_failed : Outport
  debouncevalue_for_passed : Outport  Port=2
  failed : Outport  Port=3
  passed : Outport  Port=4
  wires:
  AEMS_DEM_TIME_BASED_DEBOUNCE_THRSHOLD_DYN_CALL3/4(passed) -> Mux4/3
  AEMS_DEM_TIME_BASED_DEBOUNCE_THRSHOLD_DYN_CALL3/3(failed) -> Mux3/3
  AEMS_DEM_TIME_BASED_DEBOUNCE_THRSHOLD_DYN_CALL3/2(debouncevalue_for_passed) -> Mux2/3
  AEMS_DEM_TIME_BASED_DEBOUNCE_THRSHOLD_DYN_CALL3/1(debouncevalue_for_failed) -> Mux1/3
  Demux7/3 -> AEMS_DEM_TIME_BASED_DEBOUNCE_THRSHOLD_DYN_CALL3/7(DemCounterPassedThreshold)
  Demux6/3 -> AEMS_DEM_TIME_BASED_DEBOUNCE_THRSHOLD_DYN_CALL3/6(DemCounterFailedThreshold)
  Demux5/3 -> AEMS_DEM_TIME_BASED_DEBOUNCE_THRSHOLD_DYN_CALL3/5(DemDebounceBehavior)
  Demux4/3 -> AEMS_DEM_TIME_BASED_DEBOUNCE_THRSHOLD_DYN_CALL3/4(reseteventdebounce)
  Demux3/3 -> AEMS_DEM_TIME_BASED_DEBOUNCE_THRSHOLD_DYN_CALL3/3(prepassed)
  Demux2/3 -> AEMS_DEM_TIME_BASED_DEBOUNCE_THRSHOLD_DYN_CALL3/2(prefailed)
  Demux1/3 -> AEMS_DEM_TIME_BASED_DEBOUNCE_THRSHOLD_DYN_CALL3/1(conditionfulfilled)
  Demux/3 -> AEMS_DEM_TIME_BASED_DEBOUNCE_THRSHOLD_DYN_CALL3/Enable
  AEMS_DEM_TIME_BASED_DEBOUNCE_THRSHOLD_DYN_CALL2/4(passed) -> Mux4/2
  Mux4/1 -> passed/1
  AEMS_DEM_TIME_BASED_DEBOUNCE_THRSHOLD_DYN_CALL1/4(passed) -> Mux4/1
  AEMS_DEM_TIME_BASED_DEBOUNCE_THRSHOLD_DYN_CALL2/3(failed) -> Mux3/2
  AEMS_DEM_TIME_BASED_DEBOUNCE_THRSHOLD_DYN_CALL1/3(failed) -> Mux3/1
  Mux3/1 -> failed/1
  AEMS_DEM_TIME_BASED_DEBOUNCE_THRSHOLD_DYN_CALL2/2(debouncevalue_for_passed) -> Mux2/2
  AEMS_DEM_TIME_BASED_DEBOUNCE_THRSHOLD_DYN_CALL1/2(debouncevalue_for_passed) -> Mux2/1
  Mux2/1 -> debouncevalue_for_passed/1
  AEMS_DEM_TIME_BASED_DEBOUNCE_THRSHOLD_DYN_CALL2/1(debouncevalue_for_failed) -> Mux1/2
  AEMS_DEM_TIME_BASED_DEBOUNCE_THRSHOLD_DYN_CALL1/1(debouncevalue_for_failed) -> Mux1/1
  Mux1/1 -> debouncevalue_for_failed/1
  Demux7/2 -> AEMS_DEM_TIME_BASED_DEBOUNCE_THRSHOLD_DYN_CALL2/7(DemCounterPassedThreshold)
  passedthreshold/1 -> Demux7/1  "passedthreshold"
  Demux7/1 -> AEMS_DEM_TIME_BASED_DEBOUNCE_THRSHOLD_DYN_CALL1/7(DemCounterPassedThreshold)
  Demux6/2 -> AEMS_DEM_TIME_BASED_DEBOUNCE_THRSHOLD_DYN_CALL2/6(DemCounterFailedThreshold)
  failedthreshold/1 -> Demux6/1  "failedthreshold"
  Demux6/1 -> AEMS_DEM_TIME_BASED_DEBOUNCE_THRSHOLD_DYN_CALL1/6(DemCounterFailedThreshold)
  Demux5/2 -> AEMS_DEM_TIME_BASED_DEBOUNCE_THRSHOLD_DYN_CALL2/5(DemDebounceBehavior)
  Demux5/1 -> AEMS_DEM_TIME_BASED_DEBOUNCE_THRSHOLD_DYN_CALL1/5(DemDebounceBehavior)
  DemDebounceBehavior/1 -> Demux5/1  "behavior"
  Demux4/2 -> AEMS_DEM_TIME_BASED_DEBOUNCE_THRSHOLD_DYN_CALL2/4(reseteventdebounce)
  reseteventdebounce/1 -> Demux4/1  "reseteventdebounce"
  Demux4/1 -> AEMS_DEM_TIME_BASED_DEBOUNCE_THRSHOLD_DYN_CALL1/4(reseteventdebounce)
  Demux3/2 -> AEMS_DEM_TIME_BASED_DEBOUNCE_THRSHOLD_DYN_CALL2/3(prepassed)
  Demux3/1 -> AEMS_DEM_TIME_BASED_DEBOUNCE_THRSHOLD_DYN_CALL1/3(prepassed)
  prepassed/1 -> Demux3/1  "prepassed"
  Demux2/2 -> AEMS_DEM_TIME_BASED_DEBOUNCE_THRSHOLD_DYN_CALL2/2(prefailed)
  Demux2/1 -> AEMS_DEM_TIME_BASED_DEBOUNCE_THRSHOLD_DYN_CALL1/2(prefailed)
  prefailed/1 -> Demux2/1  "prefailed"
  Demux1/2 -> AEMS_DEM_TIME_BASED_DEBOUNCE_THRSHOLD_DYN_CALL2/1(conditionfulfilled)
  Demux/2 -> AEMS_DEM_TIME_BASED_DEBOUNCE_THRSHOLD_DYN_CALL2/Enable
  Demux1/1 -> AEMS_DEM_TIME_BASED_DEBOUNCE_THRSHOLD_DYN_CALL1/1(conditionfulfilled)
  conditionfulfilled/1 -> Demux1/1  "conditionfulfilled"
  Demux/1 -> AEMS_DEM_TIME_BASED_DEBOUNCE_THRSHOLD_DYN_CALL1/Enable
  flag_set/1 -> Demux/1

== system AEMS_Standard_Library/SUB/AEMS_DEM_TIME_BASED_DEBOUNCE_THRSHOLD_DYN_4D ==
  note: DemDebounceBehavior
  flag_set : Inport
  conditionfulfilled : Inport  Port=2
  prefailed : Inport  Port=3
  prepassed : Inport  Port=4
  reseteventdebounce : Inport  Port=5
  failedthreshold : Inport  Port=6
  passedthreshold : Inport  Port=7
  AEMS_DEM_TIME_BASED_DEBOUNCE_THRSHOLD_DYN_CALL1 : Subsystem
  AEMS_DEM_TIME_BASED_DEBOUNCE_THRSHOLD_DYN_CALL2 : Subsystem
  AEMS_DEM_TIME_BASED_DEBOUNCE_THRSHOLD_DYN_CALL3 : Subsystem
  AEMS_DEM_TIME_BASED_DEBOUNCE_THRSHOLD_DYN_CALL4 : Subsystem
  DemDebounceBehavior : Constant  Value=[0,0,0,0]  OutDataTypeStr=uint8
  Demux{,1..7} (8 alike) : Demux
  Mux{1..4} (4 alike) : Mux
  debouncevalue_for_failed : Outport
  debouncevalue_for_passed : Outport  Port=2
  failed : Outport  Port=3
  passed : Outport  Port=4
  wires:
  AEMS_DEM_TIME_BASED_DEBOUNCE_THRSHOLD_DYN_CALL4/4(passed) -> Mux4/4
  AEMS_DEM_TIME_BASED_DEBOUNCE_THRSHOLD_DYN_CALL4/3(failed) -> Mux3/4
  AEMS_DEM_TIME_BASED_DEBOUNCE_THRSHOLD_DYN_CALL4/2(debouncevalue_for_passed) -> Mux2/4
  AEMS_DEM_TIME_BASED_DEBOUNCE_THRSHOLD_DYN_CALL4/1(debouncevalue_for_failed) -> Mux1/4
  Demux7/4 -> AEMS_DEM_TIME_BASED_DEBOUNCE_THRSHOLD_DYN_CALL4/7(DemCounterPassedThreshold)
  Demux6/4 -> AEMS_DEM_TIME_BASED_DEBOUNCE_THRSHOLD_DYN_CALL4/6(DemCounterFailedThreshold)
  Demux5/4 -> AEMS_DEM_TIME_BASED_DEBOUNCE_THRSHOLD_DYN_CALL4/5(DemDebounceBehavior)
  Demux4/4 -> AEMS_DEM_TIME_BASED_DEBOUNCE_THRSHOLD_DYN_CALL4/4(reseteventdebounce)
  Demux3/4 -> AEMS_DEM_TIME_BASED_DEBOUNCE_THRSHOLD_DYN_CALL4/3(prepassed)
  Demux2/4 -> AEMS_DEM_TIME_BASED_DEBOUNCE_THRSHOLD_DYN_CALL4/2(prefailed)
  Demux1/4 -> AEMS_DEM_TIME_BASED_DEBOUNCE_THRSHOLD_DYN_CALL4/1(conditionfulfilled)
  Demux/4 -> AEMS_DEM_TIME_BASED_DEBOUNCE_THRSHOLD_DYN_CALL4/Enable
  AEMS_DEM_TIME_BASED_DEBOUNCE_THRSHOLD_DYN_CALL3/4(passed) -> Mux4/3
  AEMS_DEM_TIME_BASED_DEBOUNCE_THRSHOLD_DYN_CALL3/3(failed) -> Mux3/3
  AEMS_DEM_TIME_BASED_DEBOUNCE_THRSHOLD_DYN_CALL3/2(debouncevalue_for_passed) -> Mux2/3
  AEMS_DEM_TIME_BASED_DEBOUNCE_THRSHOLD_DYN_CALL3/1(debouncevalue_for_failed) -> Mux1/3
  Demux7/3 -> AEMS_DEM_TIME_BASED_DEBOUNCE_THRSHOLD_DYN_CALL3/7(DemCounterPassedThreshold)
  Demux6/3 -> AEMS_DEM_TIME_BASED_DEBOUNCE_THRSHOLD_DYN_CALL3/6(DemCounterFailedThreshold)
  Demux5/3 -> AEMS_DEM_TIME_BASED_DEBOUNCE_THRSHOLD_DYN_CALL3/5(DemDebounceBehavior)
  Demux4/3 -> AEMS_DEM_TIME_BASED_DEBOUNCE_THRSHOLD_DYN_CALL3/4(reseteventdebounce)
  Demux3/3 -> AEMS_DEM_TIME_BASED_DEBOUNCE_THRSHOLD_DYN_CALL3/3(prepassed)
  Demux2/3 -> AEMS_DEM_TIME_BASED_DEBOUNCE_THRSHOLD_DYN_CALL3/2(prefailed)
  Demux1/3 -> AEMS_DEM_TIME_BASED_DEBOUNCE_THRSHOLD_DYN_CALL3/1(conditionfulfilled)
  Demux/3 -> AEMS_DEM_TIME_BASED_DEBOUNCE_THRSHOLD_DYN_CALL3/Enable
  AEMS_DEM_TIME_BASED_DEBOUNCE_THRSHOLD_DYN_CALL2/4(passed) -> Mux4/2
  Mux4/1 -> passed/1
  AEMS_DEM_TIME_BASED_DEBOUNCE_THRSHOLD_DYN_CALL1/4(passed) -> Mux4/1
  AEMS_DEM_TIME_BASED_DEBOUNCE_THRSHOLD_DYN_CALL2/3(failed) -> Mux3/2
  AEMS_DEM_TIME_BASED_DEBOUNCE_THRSHOLD_DYN_CALL1/3(failed) -> Mux3/1
  Mux3/1 -> failed/1
  AEMS_DEM_TIME_BASED_DEBOUNCE_THRSHOLD_DYN_CALL2/2(debouncevalue_for_passed) -> Mux2/2
  AEMS_DEM_TIME_BASED_DEBOUNCE_THRSHOLD_DYN_CALL1/2(debouncevalue_for_passed) -> Mux2/1
  Mux2/1 -> debouncevalue_for_passed/1
  AEMS_DEM_TIME_BASED_DEBOUNCE_THRSHOLD_DYN_CALL2/1(debouncevalue_for_failed) -> Mux1/2
  AEMS_DEM_TIME_BASED_DEBOUNCE_THRSHOLD_DYN_CALL1/1(debouncevalue_for_failed) -> Mux1/1
  Mux1/1 -> debouncevalue_for_failed/1
  Demux7/2 -> AEMS_DEM_TIME_BASED_DEBOUNCE_THRSHOLD_DYN_CALL2/7(DemCounterPassedThreshold)
  passedthreshold/1 -> Demux7/1  "passedthreshold"
  Demux7/1 -> AEMS_DEM_TIME_BASED_DEBOUNCE_THRSHOLD_DYN_CALL1/7(DemCounterPassedThreshold)
  Demux6/2 -> AEMS_DEM_TIME_BASED_DEBOUNCE_THRSHOLD_DYN_CALL2/6(DemCounterFailedThreshold)
  failedthreshold/1 -> Demux6/1  "failedthreshold"
  Demux6/1 -> AEMS_DEM_TIME_BASED_DEBOUNCE_THRSHOLD_DYN_CALL1/6(DemCounterFailedThreshold)
  Demux5/2 -> AEMS_DEM_TIME_BASED_DEBOUNCE_THRSHOLD_DYN_CALL2/5(DemDebounceBehavior)
  Demux5/1 -> AEMS_DEM_TIME_BASED_DEBOUNCE_THRSHOLD_DYN_CALL1/5(DemDebounceBehavior)
  DemDebounceBehavior/1 -> Demux5/1  "behavior"
  Demux4/2 -> AEMS_DEM_TIME_BASED_DEBOUNCE_THRSHOLD_DYN_CALL2/4(reseteventdebounce)
  reseteventdebounce/1 -> Demux4/1  "reseteventdebounce"
  Demux4/1 -> AEMS_DEM_TIME_BASED_DEBOUNCE_THRSHOLD_DYN_CALL1/4(reseteventdebounce)
  Demux3/2 -> AEMS_DEM_TIME_BASED_DEBOUNCE_THRSHOLD_DYN_CALL2/3(prepassed)
  Demux3/1 -> AEMS_DEM_TIME_BASED_DEBOUNCE_THRSHOLD_DYN_CALL1/3(prepassed)
  prepassed/1 -> Demux3/1  "prepassed"
  Demux2/2 -> AEMS_DEM_TIME_BASED_DEBOUNCE_THRSHOLD_DYN_CALL2/2(prefailed)
  Demux2/1 -> AEMS_DEM_TIME_BASED_DEBOUNCE_THRSHOLD_DYN_CALL1/2(prefailed)
  prefailed/1 -> Demux2/1  "prefailed"
  Demux1/2 -> AEMS_DEM_TIME_BASED_DEBOUNCE_THRSHOLD_DYN_CALL2/1(conditionfulfilled)
  Demux/2 -> AEMS_DEM_TIME_BASED_DEBOUNCE_THRSHOLD_DYN_CALL2/Enable
  Demux1/1 -> AEMS_DEM_TIME_BASED_DEBOUNCE_THRSHOLD_DYN_CALL1/1(conditionfulfilled)
  conditionfulfilled/1 -> Demux1/1  "conditionfulfilled"
  Demux/1 -> AEMS_DEM_TIME_BASED_DEBOUNCE_THRSHOLD_DYN_CALL1/Enable
  flag_set/1 -> Demux/1
